simulink model "banka"  (R2016b)
settings: Solver=VariableStepAuto  StartTime=0.0  StopTime=10.0  RelTol=1e-3
undefined symbols (not defined in the file): mdaadlink6208
settings Model: Creator=lenovo  LastModifiedBy=15751

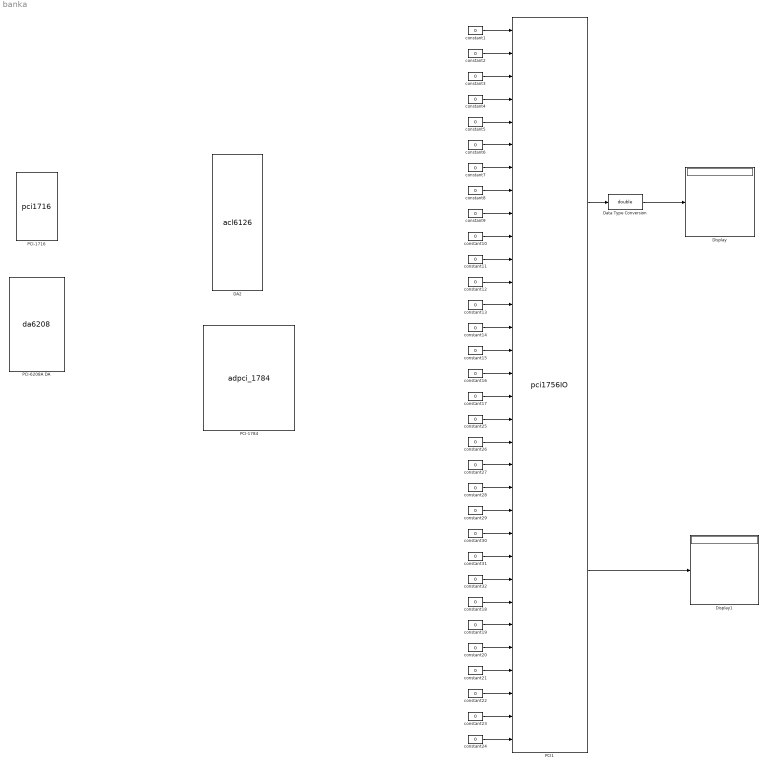
== system banka ==
  DA2 : S-Function  FunctionName=acl6126  Parameters=convBaseAddr,Range,[SampleTime SampleOffset]  SFunctionDeploymentMode=off  EnableBusSupport=off  mask(ACL-6126){sBaseAddr=0x2c0, Ranges=-10, sample=0.001}
      mask prompts: sBaseAddr "Base Address:"; sample "Sample Time:"
      mask help:
      | ACL-6126
      | HIT
      | Analog Output
      mask init:
      | convBaseAddr = 512;Range=10;SampleTime = 0.001; SampleOffset = 0;
      | sampleLength = length (sample);
      | if (sampleLength == 2)
      |   SampleTime = sample(1);
      |   SampleOffset = sample(2);
      | else
      |   SampleTime = sample(1);
      |   SampleOffset = 0;
      | end
      | 
      | sBaseAddr(find(sBaseAddr=='''')) = [];
      | index = findstr(lower(sBaseAddr),'0x');
      | if ~isempty(index) & index==1
      |   BaseAddr = sBaseAddr(3:end);
      |   baLength = length (BaseAddr);
      |   baseStringMember = [abs('0'):abs('9'),abs('a'):abs('f'),abs('A'):abs('F')];
      |   for i = 1:baLength
      |  %   if ~ismember(BaseAddr(i),baseStringMember)
      |  %     error ('Invalid character in hexadecimal string');
      |  %   end
      |   end
      |   convBaseAddr = hex2dec(BaseAddr);
      | else
      |   convBaseAddr = str2num(BaseAddr);
      |   end
      |  Range=Ranges;
      mask Help: helpview([docroot '/toolbox/xpc/pt_io_block_reference.html#xpcioref'])
      mask Display:
      | disp('ACL-6126\ncumt\nAnalog Output');
      | port_label('input',1 , '1');
      | port_label('input',2 , '2');
      | port_label('input',3 , '3');
      | port_label('input',4 , '4');
      | port_label('input',5, '5');
      | port_label('input',6 , '6');
  Data Type Conversion : DataTypeConversion  OutDataTypeStr=double
  Display : Display
  Display1 : Display
  PCI-1716 : S-Function  FunctionName=pci1716  Parameters=[SampleTime SampleOffset], SLOT  SFunctionDeploymentMode=off  EnableBusSupport=off  mask(hitad3){Sample=0.001, SLOT=-1}
      mask prompts: Sample "Sample Time:"
      mask help:
      | PCi1716
      | A/D Card
      | Developed by ZhaoJinsong
      | 2012.06.02
      mask init:
      | SampleTime = 0.001; SampleOffset=0;
      mask Help: helpview([docroot '/toolbox/xpc/pt_io_block_reference.html#xpcioref'])
      mask Display:
      | disp('PCI1716  ');
      | 
      | port_label('output',1 , 'OUT');
  PCI-1784 : S-Function  FunctionName=adpci_1784  Parameters=channel, sampletime, slot  SFunctionDeploymentMode=off  EnableBusSupport=off  mask(PCI-1784){channel=[1 2 3 4 5 6 7 8], sampletime=0.002, slot=[3 7]}
      mask prompts: channel "Channel vector:"; sampletime "Sample time:"; slot "PCI slot:"
      mask help:
      | YANHUA
      | PCI-1784
      | Motor Counter
      | UESTC
      mask init:
      | [maskdisplay] = mCntPCI_1784(channel, slot);
      | set_param( gcb, 'MaskDisplay', maskdisplay );
      settings: CopyFcn=|
      | if ~strcmp(get_param(gcb,'Linkstatus'),'none') && ...
      | ~strcmp(get_param(gcb,'Linkstatus'),'implicit')
      |   set_param(gcb,'LinkStatus','none');
      | end
      mask Display: disp('PCI-1784\nUESTC\nMotor Counter');port_label('output',1,'Cnt1');port_label('output',2,'Cnt2');port_label('output',3,'Cnt3');port_label('output',4,'Cnt4');port_label('output',5,'Index1');port_label('output',6,'Index2');port_label('output',7,'Index3');port_label('output',8,'Index4');
  "PCI-6208A DA " : S-Function  InitFcn=mdaadlink6208( 1 );  FunctionName=da6208  Parameters=channel, range, sampletime, pcislot, reset, initval  SFunctionDeploymentMode=off  EnableBusSupport=off  mask(da6208){channel=[1:8], range=4 to 20 ma, reset=[0], initval=[0], sampletime=0.001, pcislot=-1}
      mask prompts: channel "Channel vector:"; reset "Reset vector:"; initval "Initial value vector:"; sampletime "Sample time:"; pcislot "PCI slot (-1: autosearch):"
      mask help:
      | PCI-6208A
      | Adlink
      | Analog Output
      mask init:
      | [maskdisplay, reset, initval]= mdaadlink6208(2, channel, reset, initval, pcislot);
      | set_param(gcb,'MaskDisplay',maskdisplay);
      mask Help: helpview(fullfile(docroot, 'mapfiles', 'xpc.map'), 'Adlink_6208A_DA')
      mask TypeOptions range: 0 to 20 ma | 5 to 25 ma | 4 to 20 ma
      mask Display: disp('PCI-6208A\nAdlink\nAnalog Output');port_label('input',1,'1');port_label('input',2,'2');port_label('input',3,'3');port_label('input',4,'4');port_label('input',5,'5');port_label('input',6,'6');port_label('input',7,'7');port_label('input',8,'8');
  PCI1 : S-Function  FunctionName=pci1756IO  Parameters=[SampleTime SampleOffset], SLOT  SFunctionDeploymentMode=off  EnableBusSupport=off  mask(PCI1756){Sample=0.002, SLOT=[2 13]}
      mask prompts: Sample "Sample time:"
      mask help:
      | PCI-1756
      | Advantech
      | Digital Input&Output
      mask init:
      | SampleTime =0.002; SampleOffset=0;
      mask Display:
      | disp('PCI1756\nDigital output&input\n');
      | port_label('input',1,'DO1');
      | port_label('input',2,'DO2');
      | port_label('input',3,'DO3');
      | port_label('input',4,'DO4');
      | port_label('input',5,'DO5');
      | port_label('input',6,'DO6');
      | port_label('input',7,'DO7');
      | port_label('input',8,'DO8');
      | port_label('input',9,'DO9');
      | port_label('input',10,'DO10');
      | port_label('input',11,'DO11');
      | port_label('input',12,'DO12');
      | port_label('input',13,'DO13');
      | port_label('input',14,'DO14');
      | port_label('input',15,'DO15');
      | port_label('input',16,'DO16');
      | port_label('input',17,'DO17');
      | port_label('input',18,'DO18');
      | port_label('input',19,'DO19');
      | port_label('input',20,'DO20');
      | port_label('input',21,'DO21');
      | port_label('input',22,'DO22');
      | port_label('input',23,'DO23');
      | port_label('input',24,'DO24');
      | port_label('input',25,'DO25');
      | port_label('input',26,'DO26');
      | port_label('input',27,'DO27');
      | port_label('input',28,'DO28');
      | port_label('input',29,'DO29');
      | port_label('input',30,'DO30');
      | port_label('input',31,'DO31');
      | port_label('input',32,'DO32');
      | port_label('output',1,'DI1');
      | port_label('output',2,'DI2');
  constant{1..32} (32 alike) : Constant  Value=0
      settings: OpenFcn=|
      | if get_param(gcb,'value')=='1',
      | set_param(gcb,'value','0');
      | else
      | set_param(gcb,'value','1');end
  wires:
  constant2/1 -> PCI1/2
  constant3/1 -> PCI1/3
  constant4/1 -> PCI1/4
  constant5/1 -> PCI1/5
  constant6/1 -> PCI1/6
  constant7/1 -> PCI1/7
  constant8/1 -> PCI1/8
  constant9/1 -> PCI1/9
  constant10/1 -> PCI1/10
  constant11/1 -> PCI1/11
  constant12/1 -> PCI1/12
  constant13/1 -> PCI1/13
  constant14/1 -> PCI1/14
  constant15/1 -> PCI1/15
  constant16/1 -> PCI1/16
  constant17/1 -> PCI1/17
  constant25/1 -> PCI1/18
  constant26/1 -> PCI1/19
  constant27/1 -> PCI1/20
  constant28/1 -> PCI1/21
  constant29/1 -> PCI1/22
  constant30/1 -> PCI1/23
  constant31/1 -> PCI1/24
  constant32/1 -> PCI1/25
  constant18/1 -> PCI1/26
  constant19/1 -> PCI1/27
  constant20/1 -> PCI1/28
  constant21/1 -> PCI1/29
  constant22/1 -> PCI1/30
  constant23/1 -> PCI1/31
  constant24/1 -> PCI1/32
  constant1/1 -> PCI1/1
  PCI1/2 -> Display1/1
  Data Type Conversion/1 -> Display/1
  PCI1/1 -> Data Type Conversion/1
